simulink model "ESP_RTW"  (Simulink 8.7)
settings: Solver=ode1  SolverMode=SingleTasking  StartTime=0.0  StopTime=inf  FixedStep=0.001  RelTol=1e-3
PreLoadFcn:
  | vehicle = 'Car'; if ~length(which('cmcmd')), cmenv; end
  | ESP_RTW_bus
  | ESP_RTW_params
InitFcn:
  | vehicle = 'Car'; if ~length(which('cmcmd')), cmenv; end
  | ESP_RTW_bus
  | ESP_RTW_params
undefined symbols (not defined in the file or in its folder): Area_Front, Area_Rear, ay_max_off, ay_max_on, ay_per_mu_max_off, ay_per_mu_max_on, Brake_ratio, brake_valve_ctrl_kP, cat1mode1_higher, cat1mode1_lower, cat1mode2_higher, cat1mode2_lower, cat1mode3_higher, cat1mode3_lower, cat2mode1_higher, cat2mode1_lower, cat2mode2_higher, cat2mode2_lower, cat2mode3_higher, cat2mode3_lower, delta_vel, diff_lock_fac, diff_lock_off, diff_lock_on, ESP_ctrl_kD, ESP_ctrl_kI, ESP_ctrl_kP, ESP_ctrl_restore_kI, ESP_min_throttle_fac, f_ax, f_slip, g, higherlimit_highvel, higherlimit_lowvel, highervel_fac, highervelocity_fac, InitialConditionForIntegrator, limit_acc, limit_selectlow, limit_starting, limit_vdiff, locktime_throttle, lowerlimit_highvel, lowerlimit_lowvel, lowervel_fac, lowervelocity_fac, min_throttle, MPS2KMPH, MSR_ctrl_kD, MSR_ctrl_kI, MSR_ctrl_kP, MSR_min_throttle_fac, PID_kD_sideslip, PID_kD_yawrate, PID_kI_sideslip, PID_kI_yawrate, PID_kP_sideslip, PID_kP_yawrate, RADpS2RpM, rBrake ... (+37)
libraries: CarMaker4SL x133, simulink x47, simulink_extras x6
(part 1 of 4)
Description:
  | CarMaker Plug-in Model Target
settings Model: Creator=IPG  LastModifiedBy=IPG
settings DataIOCC: SignalLoggingSaveFormat=ModelDataLogs
settings OptimizationCC: ExpressionDepthLimit=2147483647
settings DebuggingCC: FcnCallInpInsideContextMsg=UseLocalSettings  StateNameClashWarn=warning
settings HardwareCC: TargetHWDeviceType=32-bit Generic  ProdEqTarget=off
settings RTWCC: SystemTargetFile=CarMaker.tlc  TemplateMakefile=CarMaker_unix-win64.tmf  Description=CarMaker Plug-in Model Target
settings CodeAppCC: MaxIdLength=63
settings STFCustomTargetCC: ModelReferenceCompliant=off  GeneratePreprocessorConditionals=Disable all  MultiInstanceERTCode=on  CodeInterfacePackaging=Reusable function  CPPClassGenCompliant=on  GRTInterface=off  GenerateAllocFcn=on  SystemTargetFile=CarMaker.tlc
settings GRTTargetCC: ModelReferenceCompliant=off  ParMdlRefBuildCompliant=off  CompOptLevelCompliant=off  ConcurrentExecutionCompliant=off  CombineOutputUpdateFcns=off  MatFileLogging=off  MultiInstanceERTCode=on  CodeInterfacePackaging=Reusable function  GenerateAllocFcn=on  UseToolchainInfoCompliant=off  ExtModeMexFile=noextcomm  RTWCAPISignals=on  RTWCAPIParams=on
settings CustomProperty: DataType=string  Value=..
settings EnumStrPairs: String=Car

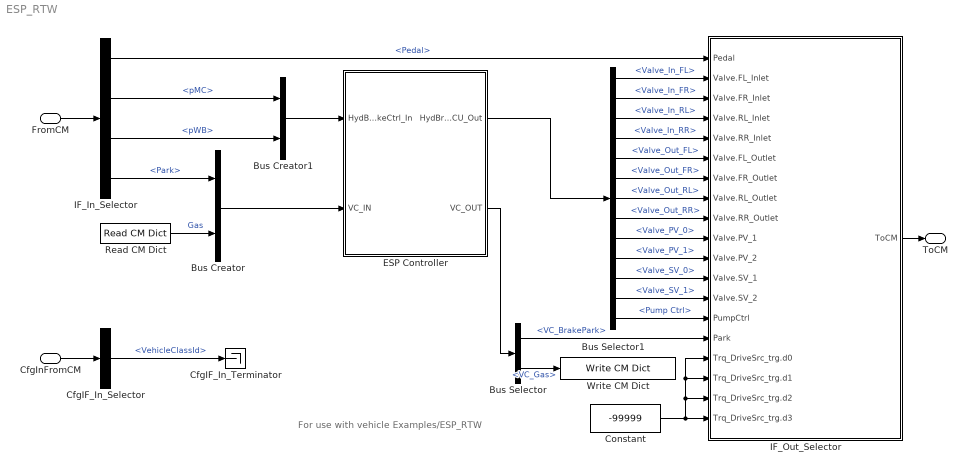
== system ESP_RTW ==
  note: For use with vehicle Examples/ESP_RTW
  FromCM : Inport  OutDataTypeStr=Bus: cmHydBrakeControlIn
  CfgInFromCM : Inport  Port=2  OutDataTypeStr=Bus: cmHydBrakeControlCfgIn
  Bus Creator : BusCreator  Inputs=2
  Bus Creator1 : BusCreator  Inputs=2
  Bus Selector : BusSelector  OutputSignals=VC_BrakePark,VC_Gas
  Bus Selector1 : BusSelector  OutputSignals=Brake Valves.Valve_In_FL,Brake Valves.Valve_In_FR,Brake Valves.Valve_In_RL,Brake Valves.Valve_In_RR,Brake Valves.Valve_Out_FL,Brake Valves.Valve_Out_FR,Brake Valves.Valve_Out_RL,Brake Valves.Valve_Out_RR,Pilot Valves.Valve_PV_0,Pilot Valves.Valve_PV_1,Suction Valves.Valve_SV_0,Suction Valves.Valve_SV_1,Pump Ctrl
  CfgIF_In_Selector : BusSelector  OutputSignals=VehicleClassId
  CfgIF_In_Terminator : Terminator
  Constant : Constant  Value=-99999
  ESP Controller : Subsystem  TreatAsAtomicUnit=on
  IF_In_Selector : BusSelector  OutputSignals=Pedal,pMC,pWB,Park
  IF_Out_Selector : Subsystem  mask(Signal Selection){}
      mask help: Signal Selection Block
      settings: OpenFcn=cmSignalSelect('SignalSelection_CB',gcb)
  Read CM Dict : CarMaker4SL/Read CM Dict  xname=VC.Gas  xsync=off
  Write CM Dict : CarMaker4SL/Write CM Dict  xname=PT.ECU.Load_lim_max  xsync=off
  ToCM : Outport  OutDataTypeStr=Bus: cmHydBrakeControlOut
  wires:
  FromCM/1 -> IF_In_Selector/1
  IF_Out_Selector/1(ToCM) -> ToCM/1
  CfgInFromCM/1 -> CfgIF_In_Selector/1
  CfgIF_In_Selector/1 -> CfgIF_In_Terminator/1  "<VehicleClassId>"
  IF_In_Selector/1 -> IF_Out_Selector/1(Pedal)  "<Pedal>"
  Bus Creator/1 -> ESP Controller/2(VC_IN)
  Bus Selector/2 -> Write CM Dict/1  "<VC_Gas>"
  Bus Selector/1 -> IF_Out_Selector/15(Park)  "<VC_BrakePark>"
  Read CM Dict/1 -> Bus Creator/2  "Gas"
  IF_In_Selector/4 -> Bus Creator/1  "<Park>"
  Bus Selector1/1 -> IF_Out_Selector/2(Valve.FL_Inlet)  "<Valve_In_FL>"
  Bus Selector1/2 -> IF_Out_Selector/3(Valve.FR_Inlet)  "<Valve_In_FR>"
  Bus Selector1/3 -> IF_Out_Selector/4(Valve.RL_Inlet)  "<Valve_In_RL>"
  Bus Selector1/4 -> IF_Out_Selector/5(Valve.RR_Inlet)  "<Valve_In_RR>"
  Bus Selector1/5 -> IF_Out_Selector/6(Valve.FL_Outlet)  "<Valve_Out_FL>"
  Bus Selector1/6 -> IF_Out_Selector/7(Valve.FR_Outlet)  "<Valve_Out_FR>"
  Bus Selector1/7 -> IF_Out_Selector/8(Valve.RL_Outlet)  "<Valve_Out_RL>"
  Bus Selector1/8 -> IF_Out_Selector/9(Valve.RR_Outlet)  "<Valve_Out_RR>"
  Bus Selector1/9 -> IF_Out_Selector/10(Valve.PV_1)  "<Valve_PV_0>"
  Bus Selector1/10 -> IF_Out_Selector/11(Valve.PV_2)  "<Valve_PV_1>"
  Bus Selector1/11 -> IF_Out_Selector/12(Valve.SV_1)  "<Valve_SV_0>"
  Bus Selector1/12 -> IF_Out_Selector/13(Valve.SV_2)  "<Valve_SV_1>"
  Bus Selector1/13 -> IF_Out_Selector/14(PumpCtrl)  "<Pump Ctrl>"
  ESP Controller/1(HydBrakeCU_Out) -> Bus Selector1/1
  ESP Controller/2(VC_OUT) -> Bus Selector/1
  Bus Creator1/1 -> ESP Controller/1(HydBrakeCtrl_In)
  IF_In_Selector/2 -> Bus Creator1/1  "<pMC>"
  IF_In_Selector/3 -> Bus Creator1/2  "<pWB>"
  Constant/1 -> IF_Out_Selector/19(Trq_DriveSrc_trg.d3), IF_Out_Selector/18(Trq_DriveSrc_trg.d2), IF_Out_Selector/17(Trq_DriveSrc_trg.d1), IF_Out_Selector/16(Trq_DriveSrc_trg.d0)

== system ESP_RTW/ESP Controller ==
  HydBrakeCtrl_In : Inport
  VC_IN : Inport  Port=2
  ESP General System : Subsystem
  ESP Input Signals : Subsystem
  Ideal Input Signals : Subsystem
  Output Signals ESP : Subsystem
  User Input Signals : Subsystem
  Vehicle Input Parameter : Subsystem
  HydBrakeCU_Out : Outport
  VC_OUT : Outport  Port=2
  wires:
  Ideal Input Signals/1(Ideal_In) -> ESP General System/4(Ideal_In)
  Vehicle Input Parameter/1(Vehicle Param) -> ESP General System/3(Vehicle Input Params)
  User Input Signals/1(User_In) -> ESP General System/2(User Input Signals)
  ESP General System/2(VC_OUT) -> VC_OUT/1
  VC_IN/1 -> ESP General System/5(VC_IN)
  ESP Input Signals/1(ESP Signals) -> ESP General System/1(ESP Input Signals)
  HydBrakeCtrl_In/1 -> ESP Input Signals/1(HydBrakeCtrl_In)
  Output Signals ESP/1(HydBrakeCU_Out) -> HydBrakeCU_Out/1
  ESP General System/1(ESP Out) -> Output Signals ESP/1(ESP Out)

== system ESP_RTW/IF_Out_Selector ==
  Pedal : Inport
  Valve.FL_Inlet : Inport  Port=2
  Valve.FR_Inlet : Inport  Port=3
  Valve.RL_Inlet : Inport  Port=4
  Valve.RR_Inlet : Inport  Port=5
  Valve.FL_Outlet : Inport  Port=6
  Valve.FR_Outlet : Inport  Port=7
  Valve.RL_Outlet : Inport  Port=8
  Valve.RR_Outlet : Inport  Port=9
  Valve.PV_1 : Inport  Port=10
  Valve.PV_2 : Inport  Port=11
  Valve.SV_1 : Inport  Port=12
  Valve.SV_2 : Inport  Port=13
  PumpCtrl : Inport  Port=14
  Park : Inport  Port=15
  Trq_DriveSrc_trg.d0 : Inport  Port=16
  Trq_DriveSrc_trg.d1 : Inport  Port=17
  Trq_DriveSrc_trg.d2 : Inport  Port=18
  Trq_DriveSrc_trg.d3 : Inport  Port=19
  BooSignal : Constant  Value=0
  RateTransition : RateTransition  OutPortSampleTime=str2num(get_param(bdroot,'FixedStep'))
  Trq_BrakeReg_trg : BusCreator  Inputs=4
  Trq_BrakeReg_trg.FL : Constant  Value=0
  Trq_BrakeReg_trg.FR : Constant  Value=0
  Trq_BrakeReg_trg.RL : Constant  Value=0
  Trq_BrakeReg_trg.RR : Constant  Value=0
  Trq_DriveSrc_trg : BusCreator  Inputs=4
  Valve : BusCreator  Inputs=16
  Valve.V_{1..4} (4 alike) : Constant  Value=0
  cmHydBrakeControlOut : BusCreator  Inputs=7
  ToCM : Outport
  wires:
  Park/1 -> cmHydBrakeControlOut/2  "Park"
  PumpCtrl/1 -> cmHydBrakeControlOut/6  "PumpCtrl"
  Valve.SV_2/1 -> Valve/12  "SV_2"
  Valve.SV_1/1 -> Valve/11  "SV_1"
  Valve.PV_2/1 -> Valve/10  "PV_2"
  Valve.PV_1/1 -> Valve/9  "PV_1"
  Valve.RR_Outlet/1 -> Valve/8  "RR_Outlet"
  Valve.RL_Outlet/1 -> Valve/7  "RL_Outlet"
  Valve.FR_Outlet/1 -> Valve/6  "FR_Outlet"
  Valve.FL_Outlet/1 -> Valve/5  "FL_Outlet"
  Valve.RR_Inlet/1 -> Valve/4  "RR_Inlet"
  Valve.RL_Inlet/1 -> Valve/3  "RL_Inlet"
  Valve.FR_Inlet/1 -> Valve/2  "FR_Inlet"
  Valve.FL_Inlet/1 -> Valve/1  "FL_Inlet"
  Pedal/1 -> cmHydBrakeControlOut/1  "Pedal"
  BooSignal/1 -> cmHydBrakeControlOut/7  "BooSignal"
  Valve.V_4/1 -> Valve/16  "V_4"
  Valve.V_3/1 -> Valve/15  "V_3"
  Valve.V_2/1 -> Valve/14  "V_2"
  Valve.V_1/1 -> Valve/13  "V_1"
  Valve/1 -> cmHydBrakeControlOut/5  "Valve"
  Trq_DriveSrc_trg/1 -> cmHydBrakeControlOut/4  "Trq_DriveSrc_trg"
  Trq_BrakeReg_trg.RR/1 -> Trq_BrakeReg_trg/4  "RR"
  Trq_BrakeReg_trg.RL/1 -> Trq_BrakeReg_trg/3  "RL"
  Trq_BrakeReg_trg.FR/1 -> Trq_BrakeReg_trg/2  "FR"
  Trq_BrakeReg_trg.FL/1 -> Trq_BrakeReg_trg/1  "FL"
  Trq_BrakeReg_trg/1 -> cmHydBrakeControlOut/3  "Trq_BrakeReg_trg"
  cmHydBrakeControlOut/1 -> RateTransition/1
  RateTransition/1 -> ToCM/1
  Trq_DriveSrc_trg.d0/1 -> Trq_DriveSrc_trg/1  "d0"
  Trq_DriveSrc_trg.d1/1 -> Trq_DriveSrc_trg/2  "d1"
  Trq_DriveSrc_trg.d2/1 -> Trq_DriveSrc_trg/3  "d2"
  Trq_DriveSrc_trg.d3/1 -> Trq_DriveSrc_trg/4  "d3"

== system ESP_RTW/ESP Controller/ESP General System ==
  ESP Input Signals : Inport
  User Input Signals : Inport  Port=2
  Vehicle Input Params : Inport  Port=3
  Ideal_In : Inport  Port=4
  VC_IN : Inport  Port=5
  ABS : Subsystem
  ASR : Subsystem
  Bus Creator : BusCreator  Inputs=6
  Bus Creator2 : BusCreator  Inputs=5
  Bus Creator3 : BusCreator  Inputs=6
  Bus Creator4 : BusCreator  Inputs=4
  ESP : Subsystem
  HSA : Subsystem
  Master Controller : Subsystem
  Signal Handling : Subsystem
  ESP Out : Outport
  VC_OUT : Outport  Port=2
  wires:
  HSA/2(BrakePark_Out) -> Master Controller/8(HSA Bus)  "BrakePark"
  HSA/1(HSA On) -> Master Controller/7(HSA On)
  Signal Handling/4(Signal Bus HSA) -> HSA/1(HSA Signal Bus)
  Signal Handling/3(Signal Bus ABS) -> ABS/1(ABS Signal Bus)
  Signal Handling/2(Signal Bus ASR) -> ASR/1(ASR Signal Bus)
  Signal Handling/1(Signal Bus ESP) -> ESP/1(ESP Signal Bus)
  Master Controller/7(VC_Out) -> VC_OUT/1  "VC_Out"
  Ideal_In/1 -> ASR/2(Ideal_In), ESP/2(Ideal_In), ABS/2(Ideal_In), HSA/2(Ideal_In)
  Master Controller/6(Diff_Torque) -> Bus Creator/6  "Diff_Torque"
  ASR/7(Diff_Torque) -> Bus Creator3/6  "Diff_Torque"
  Vehicle Input Params/1 -> ABS/3(Vehicle Params), ASR/3(Vehicle Params), ESP/3(Vehicle Params), Signal Handling/2(Vehicle Params)
  VC_IN/1 -> Master Controller/10(VC In)
  User Input Signals/1 -> ABS/4(User_In), ASR/4(User_In), ESP/4(User_In), Master Controller/9(User In)
  Bus Creator4/1 -> Master Controller/6(ABS Bus)  "ABS Bus"
  ABS/5(Pump Ctrl) -> Bus Creator4/4  "Pump Ctrl"
  ABS/4(Brake Valves) -> Bus Creator4/3  "Brake Valves"
  ABS/3(Suction Valves) -> Bus Creator4/2  "Suction Valves"
  ABS/2(Pilot Valves) -> Bus Creator4/1  "Pilot Valves"
  ASR/6(Gas_out) -> Bus Creator3/5  "Gas_Out"
  ASR/5(Pump Ctrl) -> Bus Creator3/4  "Pump Ctrl"
  ASR/4(Brake Valves) -> Bus Creator3/3  "Brake Valves"
  ASR/3(Suction Valves) -> Bus Creator3/2  "Suction Valves"
  ASR/2(Pilot Valves) -> Bus Creator3/1  "Pilot Valves"
  Master Controller/5(Pump Ctrl) -> Bus Creator/5  "Pump Ctrl"
  Master Controller/4(Suction Valves) -> Bus Creator/4  "Suction Valves"
  Master Controller/3(Pilot Valves) -> Bus Creator/3  "Pilot Valves"
  Master Controller/2(Brake Valves) -> Bus Creator/2  "Brake Valves"
  Master Controller/1(ECU Flags) -> Bus Creator/1  "ECU Flags"
  Bus Creator3/1 -> Master Controller/4(ASR Bus)  "ASR Bus"
  ABS/1(ABS On) -> Master Controller/5(ABS On)  "ABS On"
  ASR/1(ASR On) -> Master Controller/3(ASR On)  "ASR On"
  Bus Creator2/1 -> Master Controller/2(ESP Bus)  "ESP Bus"
  ESP/6(Gas_Out) -> Bus Creator2/5  "Gas_Out"
  ESP/5(Pump Ctrl) -> Bus Creator2/4  "Pump Ctrl"
  ESP/4(Brake Valves) -> Bus Creator2/3  "Brake Valves"
  ESP/3(Suction Valves) -> Bus Creator2/2  "Suction Valves"
  ESP/2(Pilot Valves) -> Bus Creator2/1  "Pilot Valves"
  ESP/1(ESP On) -> Master Controller/1(ESP On)  "ESP On"
  ESP Input Signals/1 -> Signal Handling/1(ESP In)
  Bus Creator/1 -> ESP Out/1

== system ESP_RTW/ESP Controller/ESP Input Signals ==
  HydBrakeCtrl_In : Inport
  " " : simulink_extras/Transformations/Radians to Degrees
  "   " : simulink_extras/Transformations/Radians to Degrees
  Bus Creator1 : BusCreator  Inputs=18
  Bus Selector : BusSelector  OutputSignals=Omega_B z,Acc_B y,Acc_B x
  Bus Selector1 : BusSelector  OutputSignals=pMC,pWB.FL,pWB.FR,pWB.RL,pWB.RR
  Car InertialSensor : CarMaker4SL/Car InertialSensor  xname=YRS
  Constant : Constant  Value=0
  Gain : Gain  Gain=100  SaturateOnIntegerOverflow=on  OutDataTypeStr=Inherit: Same as input  ParamDataTypeStr=Inherit: Same as input
  Gain{1..5,11} (6 alike) : Gain  Gain=RADpS2RpM  SaturateOnIntegerOverflow=on  OutDataTypeStr=Inherit: Same as input  ParamDataTypeStr=Inherit: Same as input
  Gain{6,9..10,12..15} (7 alike) : Gain  SaturateOnIntegerOverflow=on  OutDataTypeStr=Inherit: Same as input  ParamDataTypeStr=Inherit: Same as input
  Gain7 : Gain  Gain=1/g  SaturateOnIntegerOverflow=on  OutDataTypeStr=Inherit: Same as input  ParamDataTypeStr=Inherit: Same as input
  Gain8 : Gain  Gain=1/g  SaturateOnIntegerOverflow=on  OutDataTypeStr=Inherit: Same as input  ParamDataTypeStr=Inherit: Same as input
  Read CM Dict1 : CarMaker4SL/Read CM Dict  xname=Car.WheelSpd_FL  xsync=off
  Read CM Dict10 : CarMaker4SL/Read CM Dict  xname=PT.Clutch.rotv_out  xsync=off
  Read CM Dict11 : CarMaker4SL/Read CM Dict  xname=Steer.WhlAng  xsync=off
  Read CM Dict12 : CarMaker4SL/Read CM Dict  xname=PT.Engine.Trq  xsync=off
  Read CM Dict15 : CarMaker4SL/Read CM Dict  xname=PT.GearBox.GearNo  xsync=off
  Read CM Dict2 : CarMaker4SL/Read CM Dict  xname=Car.WheelSpd_FR  xsync=off
  Read CM Dict3 : CarMaker4SL/Read CM Dict  xname=Car.WheelSpd_RL  xsync=off
  Read CM Dict4 : CarMaker4SL/Read CM Dict  xname=Car.WheelSpd_RR  xsync=off
  Read CM Dict7 : CarMaker4SL/Read CM Dict  xname=PT.Engine.rotv  xsync=off
  Read CM Dict9 : CarMaker4SL/Read CM Dict  xname=VC.Gas  xsync=off
  Relational Operator : RelationalOperator  Operator=<  OutDataTypeStr=boolean
  Stop Simulation : Stop
  ESP Signals : Outport
  wires:
  Gain9/1 -> Bus Creator1/9  "Engine crankshaft output torque [Nm]"
  Gain13/1 -> Bus Creator1/14  "GearState [-]"
  " "/1 -> Bus Creator1/13  "Steering Wheel Angle [deg]"
  Gain11/1 -> Bus Creator1/12  "Torque Converter Speed [rpm]"
  Gain10/1 -> Bus Creator1/10  "Master Cylinder Pressure [bar]"
  Gain8/1 -> Bus Creator1/7  "Sensor Longitudinal acceleration [g]"
  Gain7/1 -> Bus Creator1/6  "Sensor Lateral acceleration [g]"
  "   "/1 -> Bus Creator1/5  "Sensor YawRate [degs]"
  Gain4/1 -> Bus Creator1/4  "WheelSpd RR [rpm]"
  Gain5/1 -> Bus Creator1/3  "WheelSpd RL [rpm]"
  Gain3/1 -> Bus Creator1/2  "WheelSpd FR [rpm]"
  Gain2/1 -> Bus Creator1/1  "WheelSpd FL [rpm]"
  Read CM Dict15/1 -> Gain13/1  "GearNumber [-]"
  Gain1/1 -> Bus Creator1/8  "Engine Speed [rpm]"
  Bus Selector/1 -> "   "/1  "<Omega_B z>"
  Bus Selector/3 -> Gain8/1  "<Acc_B x>"
  Car InertialSensor/2 -> Bus Selector/1
  Read CM Dict11/1 -> " "/1  "Steering Angle [rad]"
  Read CM Dict10/1 -> Gain11/1  "Clucth OutShaft [rad/s]"
  Read CM Dict9/1 -> Gain/1  "Accelerator pedal [-]"
  Bus Selector1/1 -> Gain10/1  "<pMC>"
  Read CM Dict1/1 -> Gain2/1  "WheelSpd FL [rad]/s]"
  Read CM Dict2/1 -> Gain3/1  "WheelSpd FR [rad/s]"
  Read CM Dict3/1 -> Gain5/1  "WheelSpd RL [rad/s]"
  Bus Selector/2 -> Gain7/1  "<Acc_B y>"
  Read CM Dict4/1 -> Gain4/1  "WheelSpd RR [rad/s]"
  Gain/1 -> Bus Creator1/11  "Throttle Valve Position [%]"
  Read CM Dict12/1 -> Gain9/1  "Engine Torque [Nm]"
  Read CM Dict7/1 -> Gain1/1  "Engine RotVel [rad/s]"
  Bus Creator1/1 -> ESP Signals/1
  Bus Selector1/5 -> Gain15/1  "<RR>"
  Bus Selector1/4 -> Gain14/1  "<RL>"
  Bus Selector1/3 -> Gain12/1  "<FR>"
  Bus Selector1/2 -> Gain6/1  "<FL>"
  Gain6/1 -> Bus Creator1/15  "Cylinder Pressure FL [bar]"
  Gain12/1 -> Bus Creator1/16  "Cylinder Pressure FR [bar]"
  Gain14/1 -> Bus Creator1/17  "Cylinder Pressure RL [bar]"
  Gain15/1 -> Bus Creator1/18  "Cylinder Pressure RR [bar]"
  Relational Operator/1 -> Stop Simulation/1
  Car InertialSensor/1 -> Relational Operator/1
  Constant/1 -> Relational Operator/2
  HydBrakeCtrl_In/1 -> Bus Selector1/1

== system ESP_RTW/ESP Controller/Ideal Input Signals ==
  Bus Creator1 : BusCreator  Inputs=8
  Bus Creator2 : BusCreator  Inputs=4
  Bus Creator3 : BusCreator  Inputs=2
  Bus Creator4 : BusCreator  Inputs=2
  Bus Creator5 : BusCreator  Inputs=3
  Bus Creator6 : BusCreator  Inputs=2
  Read CM Dict1 : CarMaker4SL/Read CM Dict  xname=Car.Pitch  xsync=off
  Read CM Dict10 : CarMaker4SL/Read CM Dict  xname=Car.FzRL  xsync=off
  Read CM Dict11 : CarMaker4SL/Read CM Dict  xname=Car.YawRate  xsync=off
  Read CM Dict13 : CarMaker4SL/Read CM Dict  xname=Car.CRL.Trq_T2W  xsync=off
  Read CM Dict14 : CarMaker4SL/Read CM Dict  xname=Car.LongSlipRL  xsync=off
  Read CM Dict16 : CarMaker4SL/Read CM Dict  xname=Car.CRR.Trq_T2W  xsync=off
  Read CM Dict17 : CarMaker4SL/Read CM Dict  xname=Car.FzRR  xsync=off
  Read CM Dict19 : CarMaker4SL/Read CM Dict  xname=Car.LongSlipRR  xsync=off
  Read CM Dict2 : CarMaker4SL/Read CM Dict  xname=Car.v  xsync=off
  Read CM Dict3 : CarMaker4SL/Read CM Dict  xname=Car.muRoadFR  xsync=off
  Read CM Dict4 : CarMaker4SL/Read CM Dict  xname=Car.muRoadRL  xsync=off
  Read CM Dict5 : CarMaker4SL/Read CM Dict  xname=Car.SideSlipAngle  xsync=off
  Read CM Dict6 : CarMaker4SL/Read CM Dict  xname=Car.muRoadFL  xsync=off
  Read CM Dict7 : CarMaker4SL/Read CM Dict  xname=Car.muRoadRR  xsync=off
  Read CM Dict8 : CarMaker4SL/Read CM Dict  xname=Car.vx  xsync=off
  Read CM Dict9 : CarMaker4SL/Read CM Dict  xname=Car.vy  xsync=off
  Ideal_In : Outport
  wires:
  Bus Creator6/1 -> Bus Creator1/8  "Ideal_Slip"
  Bus Creator4/1 -> Bus Creator1/7  "Ideal_Fz"
  Bus Creator3/1 -> Bus Creator1/6  "Idea_Trq2W"
  Bus Creator2/1 -> Bus Creator1/5  "Ideal_mu"
  Read CM Dict11/1 -> Bus Creator1/4  "Ideal_YawRate"
  Read CM Dict19/1 -> Bus Creator6/2  "Ideal_SlipRR"
  Read CM Dict14/1 -> Bus Creator6/1  "Ideal_SlipRL"
  Read CM Dict9/1 -> Bus Creator5/3  "Ideal_Velocity_y"
  Bus Creator5/1 -> Bus Creator1/2  "Ideal_Velocity"
  Read CM Dict8/1 -> Bus Creator5/2  "Ideal_Velocity_x"
  Read CM Dict2/1 -> Bus Creator5/1  "Ideal_Velocity"
  Read CM Dict5/1 -> Bus Creator1/3  "Ideal_SideSlipAngle"
  Read CM Dict1/1 -> Bus Creator1/1  "Ideal_Pitch"
  Bus Creator1/1 -> Ideal_In/1
  Read CM Dict7/1 -> Bus Creator2/4  "Ideal_muRR"
  Read CM Dict4/1 -> Bus Creator2/3  "Ideal_muRL"
  Read CM Dict3/1 -> Bus Creator2/2  "Ideal_muFR"
  Read CM Dict6/1 -> Bus Creator2/1  "Ideal_muFL"
  Read CM Dict13/1 -> Bus Creator3/1  "Ideal_Trq2WRL"
  Read CM Dict16/1 -> Bus Creator3/2  "Ideal_Trq2WRR"
  Read CM Dict10/1 -> Bus Creator4/1  "Ideal_FzRL"
  Read CM Dict17/1 -> Bus Creator4/2  "Ideal_FzRR"

== system ESP_RTW/ESP Controller/Output Signals ESP ==
  ESP Out : Inport
  Bus Creator : BusCreator  Inputs=4
  Bus Selector : BusSelector  OutputSignals=ECU Flags,Brake Valves,Pilot Valves,Suction Valves,Pump Ctrl,Diff_Torque
  Bus Selector1 : BusSelector  OutputSignals=ESP On,ASR On,ABS On,HSA On
  Bus Selector2 : BusSelector  OutputSignals=ASR On,MSR On,BMR On
  Bus Selector4 : BusSelector  OutputSignals=FrontDiff_Torque
  Data Type Conversion : DataTypeConversion
  Define CM Dict1 : CarMaker4SL/Define CM Dict  xname=ESP.ASR.MSR.active  xmono=off  xtype=Char  xdvaplace=VC  xnstates=2  xfirststate=0  xinitial=0
  Define CM Dict10 : CarMaker4SL/Define CM Dict  xname=ESP.ESP.active  xmono=off  xtype=Char  xdvaplace=VC  xnstates=2  xfirststate=0  xinitial=0
  Define CM Dict2 : CarMaker4SL/Define CM Dict  xname=ESP.ASR.BMR.active  xmono=off  xtype=Char  xdvaplace=VC  xnstates=2  xfirststate=0  xinitial=0
  Define CM Dict3 : CarMaker4SL/Define CM Dict  xname=ESP.ASR.active  xmono=off  xtype=Char  xdvaplace=VC  xnstates=2  xfirststate=0  xinitial=0
  Define CM Dict4 : CarMaker4SL/Define CM Dict  xname=ESP.HSA.active  xmono=off  xtype=Char  xdvaplace=VC  xnstates=2  xfirststate=0  xinitial=0
  Define CM Dict6 : CarMaker4SL/Define CM Dict  xname=ESP.ESP.lamp  xmono=off  xtype=Char  xdvaplace=VC  xnstates=2  xfirststate=0  xinitial=0
  Define CM Dict9 : CarMaker4SL/Define CM Dict  xname=ESP.ABS.active  xmono=off  xtype=Char  xdvaplace=VC  xnstates=2  xfirststate=0  xinitial=0
  Logical Operator : Logic  Operator=OR  AllPortsSameDT=off  OutDataTypeStr=boolean
  Read CM Dict3 : CarMaker4SL/Read CM Dict  xname=ESP.User.ESP_off  xsync=off
  Write CM Dict12 : CarMaker4SL/Write CM Dict  xname=ESP.ASR.MSR.active  xsync=off
  Write CM Dict13 : CarMaker4SL/Write CM Dict  xname=ESP.ASR.BMR.active  xsync=off
  Write CM Dict15 : CarMaker4SL/Write CM Dict  xname=ESP.ASR.active  xsync=off
  Write CM Dict17 : CarMaker4SL/Write CM Dict  xname=ESP.ABS.active  xsync=off
  Write CM Dict18 : CarMaker4SL/Write CM Dict  xname=ESP.ESP.active  xsync=off
  Write CM Dict19 : CarMaker4SL/Write CM Dict  xname=PT.Gen.DL.FDiff.DVA.Trq_A2B  xsync=off
  Write CM Dict20 : CarMaker4SL/Write CM Dict  xname=ESP.HSA.active  xsync=off
  Write CM Dict21 : CarMaker4SL/Write CM Dict  xname=ESP.ESP.lamp  xsync=off
  HydBrakeCU_Out : Outport
  wires:
  ESP Out/1 -> Bus Selector/1
  Bus Selector/1 -> Bus Selector1/1  "<ECU Flags>"
  Bus Selector1/2 -> Bus Selector2/1  "<ASR On>"
  Bus Selector1/1 -> Logical Operator/2, Write CM Dict18/1  "<ESP On>"
  Bus Selector1/3 -> Write CM Dict17/1  "<ABS On>"
  Bus Selector2/1 -> Write CM Dict15/1  "<ASR On>"
  Bus Selector2/2 -> Write CM Dict12/1  "<MSR On>"
  Bus Selector2/3 -> Write CM Dict13/1  "<BMR On>"
  Bus Selector4/1 -> Write CM Dict19/1  "<FrontDiff_Torque>"
  Bus Selector/6 -> Bus Selector4/1  "<Diff_Torque>"
  Bus Selector1/4 -> Write CM Dict20/1  "<HSA On>"
  Logical Operator/1 -> Data Type Conversion/1
  Read CM Dict3/1 -> Logical Operator/1
  Data Type Conversion/1 -> Write CM Dict21/1
  Bus Selector/2 -> Bus Creator/1  "<Brake Valves>"
  Bus Selector/3 -> Bus Creator/2  "<Pilot Valves>"
  Bus Selector/4 -> Bus Creator/3  "<Suction Valves>"
  Bus Selector/5 -> Bus Creator/4  "<Pump Ctrl>"
  Bus Creator/1 -> HydBrakeCU_Out/1

== system ESP_RTW/ESP Controller/User Input Signals ==
  note: User_Drive: 1 = Front; 2 = Rear; 3 = AllWheel
  Bus Creator1 : BusCreator  Inputs=5
  Bus Creator2 : BusCreator  Inputs=5
  Bus Creator3 : BusCreator  Inputs=2
  Bus Creator4 : BusCreator  Inputs=2
  Define CM Dict1 : CarMaker4SL/Define CM Dict  xname=ESP.User.ESP_off  xmono=off  xtype=Char  xdvaplace=IO_Out  xnstates=2  xfirststate=0  xinitial=0
  Define CM Dict10 : CarMaker4SL/Define CM Dict  xname=ESP.User.HSA_off  xmono=off  xtype=Char  xdvaplace=IO_Out  xnstates=2  xfirststate=0  xinitial=0
  Define CM Dict11 : CarMaker4SL/Define CM Dict  xname=ESP.User.oneWheel_on  xmono=off  xtype=Char  xdvaplace=IO_Out  xnstates=2  xfirststate=0  xinitial=0
  Define CM Dict2 : CarMaker4SL/Define CM Dict  xname=ESP.User.ASR_off  xmono=off  xtype=Char  xdvaplace=IO_Out  xnstates=2  xfirststate=0  xinitial=0
  Define CM Dict3 : CarMaker4SL/Define CM Dict  xname=ESP.User.ABS_off  xmono=off  xtype=Char  xdvaplace=IO_Out  xnstates=2  xfirststate=0  xinitial=0
  Define CM Dict4 : CarMaker4SL/Define CM Dict  xname=ESP.User.ESP_all_off  xmono=off  xtype=Char  xdvaplace=IO_Out  xnstates=2  xfirststate=0  xinitial=0
  Define CM Dict5 : CarMaker4SL/Define CM Dict  xname=ESP.User.Drive  xmono=off  xtype=Char  xdvaplace=IO_Out  xnstates=3  xfirststate=1  xinitial=1
  Define CM Dict6 : CarMaker4SL/Define CM Dict  xname=ESP.User.SideSlip_estimator_on  xmono=off  xtype=Char  xdvaplace=IO_Out  xnstates=2  xfirststate=0  xinitial=0
  Define CM Dict7 : CarMaker4SL/Define CM Dict  xname=ESP.User.mue_estimator_on  xmono=off  xtype=Char  xdvaplace=IO_Out  xnstates=2  xfirststate=0  xinitial=0
  Define CM Dict8 : CarMaker4SL/Define CM Dict  xname=ESP.User.DiffLockDVA_on  xmono=off  xtype=Char  xdvaplace=IO_Out  xnstates=2  xfirststate=0  xinitial=0
  Define CM Dict9 : CarMaker4SL/Define CM Dict  xname=ESP.User.DiffLockDVA_Trq  xunit=Nm  xmono=off  xtype=Double4  xdvaplace=IO_Out  xnstates=2  xfirststate=0  xinitial=0
  Read CM Dict1 : CarMaker4SL/Read CM Dict  xname=ESP.User.Drive  xsync=off
  Read CM Dict10 : CarMaker4SL/Read CM Dict  xname=ESP.User.HSA_off  xsync=off
  Read CM Dict11 : CarMaker4SL/Read CM Dict  xname=ESP.User.oneWheel_on  xsync=off
  Read CM Dict2 : CarMaker4SL/Read CM Dict  xname=ESP.User.ESP_all_off  xsync=off
  Read CM Dict3 : CarMaker4SL/Read CM Dict  xname=ESP.User.ESP_off  xsync=off
  Read CM Dict4 : CarMaker4SL/Read CM Dict  xname=ESP.User.ASR_off  xsync=off
  Read CM Dict5 : CarMaker4SL/Read CM Dict  xname=ESP.User.ABS_off  xsync=off
  Read CM Dict6 : CarMaker4SL/Read CM Dict  xname=ESP.User.SideSlip_estimator_on  xsync=off
  Read CM Dict7 : CarMaker4SL/Read CM Dict  xname=ESP.User.mue_estimator_on  xsync=off
  Read CM Dict8 : CarMaker4SL/Read CM Dict  xname=ESP.User.DiffLockDVA_on  xsync=off
  Read CM Dict9 : CarMaker4SL/Read CM Dict  xname=ESP.User.DiffLockDVA_Trq  xsync=off
  User_In : Outport
  wires:
  Read CM Dict11/1 -> Bus Creator1/5  "User_oneWheel_on"
  Read CM Dict10/1 -> Bus Creator2/5  "User_Switch_HSA_off"
  Bus Creator4/1 -> Bus Creator1/4  "User_DiffLock"
  Read CM Dict9/1 -> Bus Creator4/2  "User_DiffLock_Trq"
  Read CM Dict8/1 -> Bus Creator4/1  "User_DiffLock_on"
  Bus Creator3/1 -> Bus Creator1/3  "User_estimators_on"
  Read CM Dict7/1 -> Bus Creator3/2  "User_mue_estimator_on"
  Read CM Dict6/1 -> Bus Creator3/1  "User_SideSlip_estimator_on"
  Bus Creator2/1 -> Bus Creator1/2  "User_Switch"
  Read CM Dict2/1 -> Bus Creator2/1  "User_Switch_Main_off"
  Read CM Dict3/1 -> Bus Creator2/2  "User_Switch_ESP_off"
  Read CM Dict4/1 -> Bus Creator2/3  "User_Switch_ASR_off"
  Read CM Dict5/1 -> Bus Creator2/4  "User_Switch_ABS_off"
  Bus Creator1/1 -> User_In/1
  Read CM Dict1/1 -> Bus Creator1/1  "User_Drive"

== system ESP_RTW/ESP Controller/Vehicle Input Parameter ==
  note: Note:
      | We could also use
      | the left wheel as is has
      | the same coordinate
      | as regards x-axis
      | (which interests us here)
  note: Note:
      | We could also use
      | the left wheel as is has
      | the same coordinate
      | as regards x-axis
      | (which interests us here)
  Bus Creator{,1..3} (4 alike) : BusCreator  Inputs=4
  Bus Creator4 : BusCreator  Inputs=2
  Read CM Parameter : CarMaker4SL/Read CM Parameter  xfile=TireFL  xkey=KinRollRadius  xnout=1  xdefaults=0  xmuxed=on
  Read CM Parameter1 : CarMaker4SL/Read CM Parameter  xfile=TireFR  xkey=KinRollRadius  xnout=1  xdefaults=0  xmuxed=on
  Read CM Parameter2 : CarMaker4SL/Read CM Parameter  xfile=TireRL  xkey=KinRollRadius  xnout=1  xdefaults=0  xmuxed=on
  Read CM Parameter3 : CarMaker4SL/Read CM Parameter  xfile=TireRR  xkey=KinRollRadius  xnout=1  xdefaults=0  xmuxed=on
  Read CM Parameter4 : CarMaker4SL/Read CM Parameter  xfile=Vehicle  xkey=WheelCarrier.fr.pos  xnout=1  xdefaults=0  xmuxed=on
  Read CM Parameter5 : CarMaker4SL/Read CM Parameter  xfile=Vehicle  xkey=Body.pos  xnout=1  xdefaults=0  xmuxed=on
  Read CM Parameter6 : CarMaker4SL/Read CM Parameter  xfile=Vehicle  xkey=Body.pos  xnout=1  xdefaults=0  xmuxed=on
  Read CM Parameter7 : CarMaker4SL/Read CM Parameter  xfile=Vehicle  xkey=WheelCarrier.rr.pos  xnout=1  xdefaults=0  xmuxed=on
  Read CM Parameter8 : CarMaker4SL/Read CM Parameter  xfile=Vehicle  xkey=WheelCarrier.rl.pos  xnout=2  xdefaults=0  xmuxed=off
  Read CM Parameter9 : CarMaker4SL/Read CM Parameter  xfile=Vehicle  xkey=WheelCarrier.fl.pos  xnout=2  xdefaults=0  xmuxed=off
  Steer Angle y-Data : Constant  Value=SteerAng_Out
  Steer Wheel Angle x-Data : Constant  Value=SteerWheelAng_In
  Sum3 : Sum  Inputs=+-  SaturateOnIntegerOverflow=on  InputSameDT=on  OutDataTypeStr=Inherit: Same as first input
  Sum4 : Sum  Inputs=+-  SaturateOnIntegerOverflow=on  InputSameDT=on  OutDataTypeStr=Inherit: Same as first input
  Terminator{,1..9} (10 alike) : Terminator
  z-Position of WheelCarrier FL : CarMaker4SL/Read CM Parameter  xfile=Vehicle  xkey=WheelCarrier.fl.pos  xnout=3  xdefaults=0  xmuxed=off
  z-Position of WheelCarrier FR : CarMaker4SL/Read CM Parameter  xfile=Vehicle  xkey=WheelCarrier.fr.pos  xnout=3  xdefaults=0  xmuxed=off
  z-Position of WheelCarrier RL : CarMaker4SL/Read CM Parameter  xfile=Vehicle  xkey=WheelCarrier.rl.pos  xnout=3  xdefaults=0  xmuxed=off
  z-Position of WheelCarrier RR : CarMaker4SL/Read CM Parameter  xfile=Vehicle  xkey=WheelCarrier.rr.pos  xnout=3  xdefaults=0  xmuxed=off
  Vehicle Param : Outport
  wires:
  Bus Creator4/1 -> Bus Creator1/4  "SteeringGeometry"
  Steer Wheel Angle x-Data/1 -> Bus Creator4/1  "SteerWheelAng_In"
  Steer Angle y-Data/1 -> Bus Creator4/2  "SteerAng_Out"
  z-Position of WheelCarrier RR/2 -> Terminator9/1
  z-Position of WheelCarrier RR/1 -> Terminator8/1
  z-Position of WheelCarrier RL/2 -> Terminator7/1
  z-Position of WheelCarrier RL/1 -> Terminator6/1
  z-Position of WheelCarrier FR/2 -> Terminator5/1
  z-Position of WheelCarrier FR/1 -> Terminator4/1
  z-Position of WheelCarrier RR/3 -> Bus Creator3/4  "Param_zRR"
  z-Position of WheelCarrier RL/3 -> Bus Creator3/3  "Param_zRL"
  z-Position of WheelCarrier FR/3 -> Bus Creator3/2  "Param_zFR"
  z-Position of WheelCarrier FL/3 -> Bus Creator3/1  "Param_zFL"
  Bus Creator3/1 -> Bus Creator1/3  "CarrierGeometry"
  z-Position of WheelCarrier FL/2 -> Terminator3/1
  z-Position of WheelCarrier FL/1 -> Terminator2/1
  Read CM Parameter8/1 -> Terminator1/1
  Read CM Parameter9/1 -> Terminator/1
  Read CM Parameter9/2 -> Bus Creator2/3  "Param_bF"
  Read CM Parameter8/2 -> Bus Creator2/4  "Param_bR"
  Bus Creator2/1 -> Bus Creator1/2  "VehicleGeometry"
  Read CM Parameter6/1 -> Sum3/1
  Sum3/1 -> Bus Creator2/2  "Param_aR"
  Read CM Parameter7/1 -> Sum3/2
  Sum4/1 -> Bus Creator2/1  "Param_aF"
  Read CM Parameter4/1 -> Sum4/1
  Read CM Parameter5/1 -> Sum4/2
  Read CM Parameter2/1 -> Bus Creator/3  "Param_RadiusRL"
  Read CM Parameter/1 -> Bus Creator/1  "Param_RadiusFL"
  Bus Creator/1 -> Bus Creator1/1  "TireRadius"
  Read CM Parameter3/1 -> Bus Creator/4  "Param_RadiusRR"
  Read CM Parameter1/1 -> Bus Creator/2  "Param_RadiusFR"
  Bus Creator1/1 -> Vehicle Param/1

== system ESP_RTW/ESP Controller/ESP General System/ABS ==
  note: ABS disabled when slower than v_min
  ABS Signal Bus : Inport
  Ideal_In : Inport  Port=2
  Vehicle Params : Inport  Port=3
  User_In : Inport  Port=4
  ABS ECU : Subsystem
  Bus Creator : BusCreator  Inputs=8
  Bus Creator2 : BusCreator  Inputs=2
  Bus Creator3 : BusCreator  Inputs=2
  Bus Selector3 : BusSelector  OutputSignals=ax [m/s^2],WheelSpeeds
  Bus Selector1 : BusSelector  OutputSignals=TireRadius
  Bus Selector2 : BusSelector  OutputSignals=Param_RadiusRR,Param_RadiusRL,Param_RadiusFR,Param_RadiusFL
  Bus Selector4 : BusSelector  OutputSignals=WheelSpd_RR,WheelSpd_RL,WheelSpd_FR,WheelSpd_FL
  helpsignals estimator : Subsystem
  ABS On : Outport
  Pilot Valves : Outport  Port=2
  Suction Valves : Outport  Port=3
  Brake Valves : Outport  Port=4
  Pump Ctrl : Outport  Port=5
  wires:
  Bus Selector4/1 -> ABS ECU/9(Speed_RR)  "<WheelSpd_RR>"
  Bus Selector4/2 -> ABS ECU/8(Speed_RL)  "<WheelSpd_RL>"
  Bus Selector4/3 -> ABS ECU/7(Speed_FR)  "<WheelSpd_FR>"
  Bus Selector4/4 -> ABS ECU/6(Speed_FL)  "<WheelSpd_FL>"
  Ideal_In/1 -> helpsignals estimator/2(Ideal_In)
  Bus Selector3/1 -> helpsignals estimator/3(ax)  "<ax [m/s^2]>"
  ABS Signal Bus/1 -> Bus Selector3/1
  Bus Selector1/1 -> helpsignals estimator/5(TireRadius), Bus Selector2/1  "<TireRadius>"
  Bus Selector2/1 -> ABS ECU/13(radius_RR)  "<Param_RadiusRR>"
  Bus Selector2/2 -> ABS ECU/12(radius_RL)  "<Param_RadiusRL>"
  Bus Selector2/3 -> ABS ECU/11(radius_FR)  "<Param_RadiusFR>"
  Vehicle Params/1 -> Bus Selector1/1
  Bus Selector2/4 -> ABS ECU/10(radius_FL)  "<Param_RadiusFL>"
  User_In/1 -> helpsignals estimator/1(User_In)
  Bus Creator3/1 -> Suction Valves/1
  Bus Creator2/1 -> Pilot Valves/1
  ABS ECU/14(Valve_SV_1) -> Bus Creator3/2  "Valve_SV_1"
  ABS ECU/13(Valve_SV_0) -> Bus Creator3/1  "Valve_SV_0"
  ABS ECU/12(Valve_PV_1) -> Bus Creator2/2  "Valve_PV_1"
  ABS ECU/11(Valve_PV_0) -> Bus Creator2/1  "Valve_PV_0"
  ABS ECU/9(Brake Valve_Out_RR) -> Bus Creator/8  "Valve_Out_RR"
  ABS ECU/8(Brake Valve_Out_RL) -> Bus Creator/7  "Valve_Out_RL"
  ABS ECU/7(Brake Valve_Out_FR) -> Bus Creator/6  "Valve_Out_FR"
  ABS ECU/6(Brake Valve_Out_FL) -> Bus Creator/5  "Valve_Out_FL"
  ABS ECU/5(Brake Valve_In_RR) -> Bus Creator/4  "Valve_In_RR"
  ABS ECU/4(Brake Valve_In_RL) -> Bus Creator/3  "Valve_In_RL"
  ABS ECU/3(Brake Valve_In_FR) -> Bus Creator/2  "Valve_In_FR"
  ABS ECU/2(Brake Valve_In_FL) -> Bus Creator/1  "Valve_In_FL"
  Bus Creator/1 -> Brake Valves/1
  Bus Selector3/2 -> helpsignals estimator/4(WheelSpeeds), Bus Selector4/1  "<WheelSpeeds>"
  ABS ECU/10(ABS On) -> ABS On/1
  helpsignals estimator/5(LongSlip_RR) -> ABS ECU/5(LongSlip_RR)
  ABS ECU/1(Brake Pump Ctrl) -> Pump Ctrl/1
  helpsignals estimator/4(LongSlip_RL) -> ABS ECU/4(LongSlip_RL)
  helpsignals estimator/3(LongSlip_FR) -> ABS ECU/3(LongSlip_FR)
  helpsignals estimator/2(LongSlip_FL) -> ABS ECU/2(LongSlip_FL)
  helpsignals estimator/1(vref) -> ABS ECU/1(vref)

== system ESP_RTW/ESP Controller/ESP General System/ASR ==
  ASR Signal Bus : Inport
  Ideal_In : Inport  Port=2
  Vehicle Params : Inport  Port=3
  User_In : Inport  Port=4
  BMR ECU : Subsystem
  Bus Creator : BusCreator  Inputs=4
  Bus Creator3 : BusCreator  Inputs=3
  Bus Selector3 : BusSelector  OutputSignals=Throttle Position,WheelSpeeds
  Bus Selector : BusSelector  OutputSignals=WheelSpd_FL,WheelSpd_FR,WheelSpd_RL,WheelSpd_RR
  Bus Selector1 : BusSelector  OutputSignals=TireRadius
  Bus Selector2 : BusSelector  OutputSignals=Param_RadiusFL,Param_RadiusFR,Param_RadiusRL,Param_RadiusRR
  Constant4 : Constant  Value=MPS2KMPH
  Logical Operator2 : Logic  Operator=OR  AllPortsSameDT=off
  MSR ECU : Subsystem
  Mux1 : Mux
  Product : Product  RndMeth=Zero
  Product1 : Product  RndMeth=Zero
  ASR On : Outport
  Pilot Valves : Outport  Port=2
  Suction Valves : Outport  Port=3
  Brake Valves : Outport  Port=4
  Pump Ctrl : Outport  Port=5
  Gas_out : Outport  Port=6
  Diff_Torque : Outport  Port=7
  wires:
  Constant4/1 -> Product1/2
  Ideal_In/1 -> BMR ECU/4(Ideal_In), MSR ECU/4(Ideal_In)
  Bus Selector3/1 -> MSR ECU/1(Throttle Position), BMR ECU/1(Throttle)  "<Throttle Position>"
  ASR Signal Bus/1 -> Bus Selector3/1
  Bus Selector1/1 -> Bus Selector2/1  "<TireRadius>"
  Bus Selector2/4 -> Mux1/4  "<Param_RadiusRR>"
  Bus Selector2/3 -> Mux1/3  "<Param_RadiusRL>"
  Bus Selector2/2 -> Mux1/2  "<Param_RadiusFR>"
  Vehicle Params/1 -> Bus Selector1/1
  BMR ECU/6(Diff_Torque) -> Diff_Torque/1  "Diff_Torque"
  User_In/1 -> BMR ECU/3(User_In), MSR ECU/3(User_In)
  BMR ECU/5(Pump Ctrl) -> Pump Ctrl/1
  BMR ECU/4(Suctions Valves) -> Suction Valves/1
  BMR ECU/3(Pilot Valves) -> Pilot Valves/1
  Logical Operator2/1 -> Bus Creator3/2  "ASR On"
  Bus Creator3/1 -> ASR On/1
  MSR ECU/1(Gas_out) -> Gas_out/1
  Mux1/1 -> Product/2
  Bus Creator/1 -> Product/1
  Product1/1 -> MSR ECU/2(WheelVelocity [kmph]), BMR ECU/2(WheelVelocity [kmph])
  BMR ECU/2(Brake Valves) -> Brake Valves/1
  BMR ECU/1(BMR On) -> Bus Creator3/3, Logical Operator2/2  "BMR On"
  MSR ECU/2(MSR On) -> Logical Operator2/1, Bus Creator3/1  "MSR On"
  Bus Selector3/2 -> Bus Selector/1  "<WheelSpeeds>"
  Bus Selector2/1 -> Mux1/1  "<Param_RadiusFL>"
  Bus Selector/4 -> Bus Creator/4  "<WheelSpd_RR>"
  Bus Selector/3 -> Bus Creator/3  "<WheelSpd_RL>"
  Bus Selector/2 -> Bus Creator/2  "<WheelSpd_FR>"
  Bus Selector/1 -> Bus Creator/1  "<WheelSpd_FL>"
  Product/1 -> Product1/1

== system ESP_RTW/ESP Controller/ESP General System/ESP ==
  ESP Signal Bus : Inport
  Ideal_In : Inport  Port=2
  Vehicle Params : Inport  Port=3
  User_In : Inport  Port=4
  Actuator Brake : Subsystem
  Bus Creator : BusCreator  Inputs=8
  Bus Creator1 : BusCreator  Inputs=2
  Bus Creator2 : BusCreator  Inputs=2
  Bus Selector1 : BusSelector  OutputSignals=ax [m/s^2],Throttle Position,Yaw Rate,Steer Angle,ay [m/s^2],Wheel Cylinder Pressure
  Define CM Dict : CarMaker4SL/Define CM Dict  xname=ESP.ESP.Gas_out  xmono=off  xtype=Double4  xdvaplace=None  xnstates=0  xfirststate=0  xinitial=0
  ECU : Subsystem
  Write CM Dict : CarMaker4SL/Write CM Dict  xname=ESP.ESP.Gas_out  xsync=off
  helpsignals estimator : Subsystem
  ESP On : Outport
  Pilot Valves : Outport  Port=2
  Suction Valves : Outport  Port=3
  Brake Valves : Outport  Port=4
  Pump Ctrl : Outport  Port=5
  Gas_Out : Outport  Port=6
  wires:
  Bus Selector1/5 -> ECU/7(ay)  "<ay [m/s^2]>"
  ESP Signal Bus/1 -> Bus Selector1/1
  Vehicle Params/1 -> helpsignals estimator/3(Vehicle Params), ECU/9(Vehicle Params)
  Bus Selector1/6 -> Actuator Brake/9(Wheel Cylinder Pressure)  "<Wheel Cylinder Pressure>"
  Ideal_In/1 -> helpsignals estimator/2(Ideal_In), ECU/8(Ideal_In)
  User_In/1 -> helpsignals estimator/4(User_In), ECU/10(User_In)
  Bus Creator1/1 -> Suction Valves/1
  Bus Creator2/1 -> Pilot Valves/1
  Bus Creator/1 -> Brake Valves/1
  ECU/1(Gas_out) -> Gas_Out/1, Write CM Dict/1
  Actuator Brake/14(ESP_On) -> ESP On/1  "ESP_On"
  Actuator Brake/13(PumpCtrl) -> Pump Ctrl/1  "PumpCtrl"
  Actuator Brake/12(Valve_SV_1) -> Bus Creator1/2  "Valve_SV_1"
  Actuator Brake/11(Valve_SV_0) -> Bus Creator1/1  "Valve_SV_0"
  Actuator Brake/10(Valve_PV_1) -> Bus Creator2/2  "Valve_PV_1"
  Actuator Brake/9(Valve_PV_0) -> Bus Creator2/1  "Valve_PV_0"
  Actuator Brake/8(Valve_Out_RR) -> Bus Creator/8  "Valve_Out_RR"
  Actuator Brake/7(Valve_Out_RL) -> Bus Creator/7  "Valve_Out_RL"
  Bus Selector1/3 -> ECU/3(Yaw Rate)  "<Yaw Rate>"
  Actuator Brake/6(Valve_Out_FR) -> Bus Creator/6  "Valve_Out_FR"
  Actuator Brake/5(Valve_Out_FL) -> Bus Creator/5  "Valve_Out_FL"
  Bus Selector1/2 -> ECU/2(Throttle Position)  "<Throttle Position>"
  Actuator Brake/4(Valve_In_RR) -> Bus Creator/4  "Valve_In_RR"
  Actuator Brake/3(Valve_In_RL) -> Bus Creator/3  "Valve_In_RL"
  Bus Selector1/1 -> ECU/1(ax)  "<ax [m/s^2]>"
  Actuator Brake/2(Valve_In_FR) -> Bus Creator/2  "Valve_In_FR"
  Actuator Brake/1(Valve_In_FL) -> Bus Creator/1  "Valve_In_FL"
  Bus Selector1/4 -> helpsignals estimator/1(Steer Angle), ECU/4(Steer Angle)  "<Steer Angle>"
  helpsignals estimator/2(mu) -> ECU/6(mu)
  helpsignals estimator/1(SideslipAngle) -> ECU/5(Sideslip)
  ECU/9(RR_Trq_target) -> Actuator Brake/8(RR_Trq_target)
  ECU/8(RR_active) -> Actuator Brake/7(RR_active)
  ECU/7(RL_Trq_target) -> Actuator Brake/6(RL_Trq_target)
  ECU/6(RL_active) -> Actuator Brake/5(RL_active)
  ECU/5(FR_Trq_target) -> Actuator Brake/4(FR_Trq_target)
  ECU/4(FR_active) -> Actuator Brake/3(FR_active)
  ECU/3(FL_Trq_target) -> Actuator Brake/2(FL_Trq_target)
  ECU/2(FL_active) -> Actuator Brake/1(FL_active)

== system ESP_RTW/ESP Controller/ESP General System/HSA ==
  HSA Signal Bus : Inport
  Ideal_In : Inport  Port=2
  Bus Selector2 : BusSelector  OutputSignals=Engine crankshaft output torque [Nm]
  Bus Selector1 : BusSelector  OutputSignals=Ideal_Pitch,Ideal_Velocity.Ideal_Velocity_x
  Data Type Conversion : DataTypeConversion
  Gain : Gain  Gain=-1
  Logical Operator : Logic  Inputs=3  AllPortsSameDT=off  OutDataTypeStr=boolean
  Relay : Relay  OnSwitchValue=threshold_carpitch_on  OffSwitchValue=threshold_carpitch_off
  Relay1 : Relay  OnSwitchValue=threshold_velocity_on  OffSwitchValue=threshold_velocity_off  OnOutputValue=0  OffOutputValue=1
  Relay2 : Relay  OnSwitchValue=threshold_eng_trq_on  OffSwitchValue=threshold_eng_trq_off  OnOutputValue=0  OffOutputValue=1
  HSA On : Outport
  BrakePark_Out : Outport  Port=2
  wires:
  Bus Selector2/1 -> Relay2/1  "<Engine crankshaft output torque [Nm]>"
  HSA Signal Bus/1 -> Bus Selector2/1
  Data Type Conversion/1 -> BrakePark_Out/1, HSA On/1
  Logical Operator/1 -> Data Type Conversion/1
  Relay/1 -> Logical Operator/2
  Relay1/1 -> Logical Operator/3
  Relay2/1 -> Logical Operator/1
  Bus Selector1/2 -> Relay1/1  "<Ideal_Velocity_x>"
  Gain/1 -> Relay/1
  Bus Selector1/1 -> Gain/1  "<Ideal_Pitch>"
  Ideal_In/1 -> Bus Selector1/1

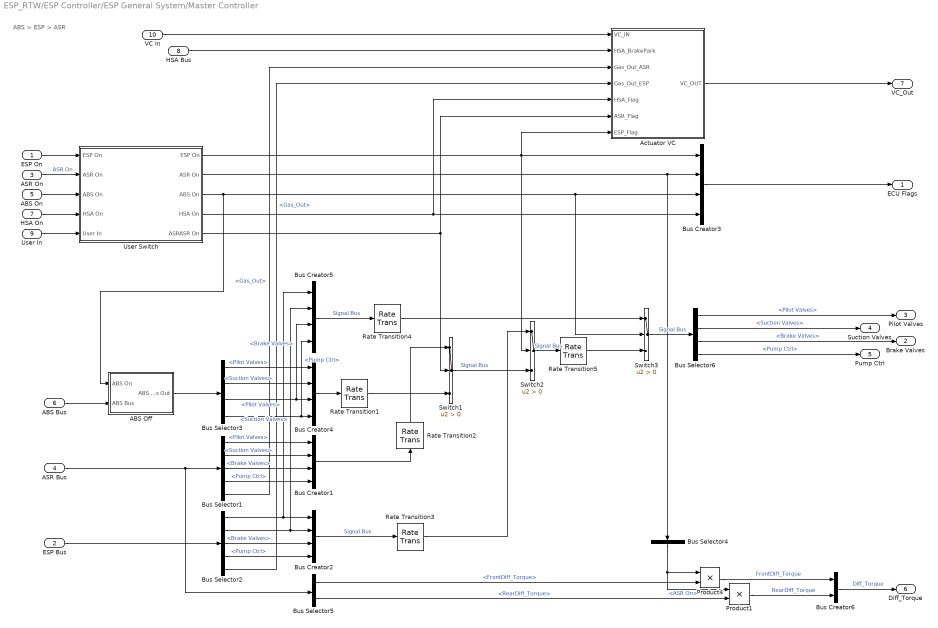
== system ESP_RTW/ESP Controller/ESP General System/Master Controller ==
  note: ABS > ESP > ASR
  ESP On : Inport
  ESP Bus : Inport  Port=2
  ASR On : Inport  Port=3
  ASR Bus : Inport  Port=4
  ABS On : Inport  Port=5
  ABS Bus : Inport  Port=6
  HSA On : Inport  Port=7
  HSA Bus : Inport  Port=8
  User In : Inport  Port=9
  VC In : Inport  Port=10
  ABS Off : Subsystem
  Actuator VC : Subsystem
  Bus Creator{1..5} (5 alike) : BusCreator  Inputs=4
  Bus Creator6 : BusCreator  Inputs=2
  Bus Selector1 : BusSelector  OutputSignals=Pilot Valves,Suction Valves,Brake Valves,Pump Ctrl,Gas_Out
  Bus Selector2 : BusSelector  OutputSignals=Pilot Valves,Suction Valves,Brake Valves,Pump Ctrl,Gas_Out
  Bus Selector3 : BusSelector  OutputSignals=Pilot Valves,Suction Valves,Brake Valves,Pump Ctrl
  Bus Selector4 : BusSelector  OutputSignals=ASR On
  Bus Selector5 : BusSelector  OutputSignals=Diff_Torque.FrontDiff_Torque,Diff_Torque.RearDiff_Torque
  Bus Selector6 : BusSelector  OutputSignals=Pilot Valves,Suction Valves,Brake Valves,Pump Ctrl
  Product1 : Product  RndMeth=Zero
  Product4 : Product  RndMeth=Zero
  Rate Transition{1..5} (5 alike) : RateTransition
  Switch1 : Switch  Criteria=u2 > Threshold
  Switch2 : Switch  Criteria=u2 > Threshold
  Switch3 : Switch  Criteria=u2 > Threshold
  User Switch : Subsystem
  ECU Flags : Outport
  Brake Valves : Outport  Port=2
  Pilot Valves : Outport  Port=3
  Suction Valves : Outport  Port=4
  Pump Ctrl : Outport  Port=5
  Diff_Torque : Outport  Port=6
  VC_Out : Outport  Port=7
  wires:
  Rate Transition5/1 -> Switch3/3
  Rate Transition4/1 -> Switch3/1
  Rate Transition3/1 -> Switch2/1
  ABS Off/1(ABS Bus Out) -> Bus Selector3/1
  Bus Selector4/1 -> Product4/1, Product1/1  "<ASR On>"
  Bus Creator6/1 -> Diff_Torque/1  "Diff_Torque"
  Product1/1 -> Bus Creator6/2  "RearDiff_Torque"
  Product4/1 -> Bus Creator6/1  "FrontDiff_Torque"
  Bus Selector5/2 -> Product1/2  "<RearDiff_Torque>"
  Bus Selector5/1 -> Product4/2  "<FrontDiff_Torque>"
  User Switch/4("HSA On ") -> Actuator VC/5(HSA_Flag), Bus Creator3/4
  HSA On/1 -> User Switch/4(HSA On)
  HSA Bus/1 -> Actuator VC/2(HSA_BrakePark)
  User Switch/2("ASR On ") -> Bus Selector4/1, Bus Creator3/2
  User In/1 -> User Switch/5(User In)
  ABS On/1 -> User Switch/3(ABS On)
  ASR On/1 -> User Switch/2(ASR On)  "ASR On"
  ESP On/1 -> User Switch/1(ESP On)
  User Switch/1("ESP On ") -> Switch2/2, Bus Creator3/1, Actuator VC/7(ESP_Flag)
  User Switch/5(ASRASR On) -> Switch1/2, Actuator VC/6(ASR_Flag)
  User Switch/3("ABS On ") -> Switch3/2, Bus Creator3/3, ABS Off/1(ABS On)
  Bus Selector2/5 -> Actuator VC/4(Gas_Out_ESP)  "<Gas_Out>"
  Bus Selector1/5 -> Actuator VC/3(Gas_Out_ASR)  "<Gas_Out>"
  Switch3/1 -> Bus Selector6/1  "Signal Bus"
  Rate Transition1/1 -> Switch1/3
  Rate Transition2/1 -> Switch1/1
  Bus Creator4/1 -> Rate Transition1/1
  Bus Creator1/1 -> Rate Transition2/1
  Bus Creator5/1 -> Rate Transition4/1  "Signal Bus"
  Switch2/1 -> Rate Transition5/1  "Signal Bus"
  Bus Selector1/4 -> Bus Creator1/4  "<Pump Ctrl>"
  Bus Selector1/3 -> Bus Creator1/3  "<Brake Valves>"
  Bus Selector1/2 -> Bus Creator1/2  "<Suction Valves>"
  Bus Selector1/1 -> Bus Creator1/1  "<Pilot Valves>"
  ASR Bus/1 -> Bus Selector1/1, Bus Selector5/1
  Bus Creator2/1 -> Rate Transition3/1  "Signal Bus"
  Switch1/1 -> Switch2/3  "Signal Bus"
  Bus Selector3/2 -> Bus Creator4/2  "<Suction Valves>"
  Bus Selector3/1 -> Bus Creator4/1  "<Pilot Valves>"
  ABS Bus/1 -> ABS Off/2(ABS Bus)
  Bus Selector3/4 -> Bus Creator4/4, Bus Creator5/4  "<Pump Ctrl>"
  Bus Selector3/3 -> Bus Creator4/3, Bus Creator5/3  "<Brake Valves>"
  Bus Selector6/4 -> Pump Ctrl/1  "<Pump Ctrl>"
  Bus Selector6/3 -> Brake Valves/1  "<Brake Valves>"
  Bus Selector6/2 -> Suction Valves/1  "<Suction Valves>"
  Bus Selector6/1 -> Pilot Valves/1  "<Pilot Valves>"
  Bus Selector2/4 -> Bus Creator2/4  "<Pump Ctrl>"
  Bus Selector2/3 -> Bus Creator2/3  "<Brake Valves>"
  Bus Selector2/2 -> Bus Creator2/2, Bus Creator5/2  "<Suction Valves>"
  Bus Selector2/1 -> Bus Creator2/1, Bus Creator5/1  "<Pilot Valves>"
  ESP Bus/1 -> Bus Selector2/1
  VC In/1 -> Actuator VC/1(VC_IN)
  Actuator VC/1(VC_OUT) -> VC_Out/1
  Bus Creator3/1 -> ECU Flags/1

== system ESP_RTW/ESP Controller/ESP General System/Signal Handling ==
  ESP In : Inport
  Vehicle Params : Inport  Port=2
  " " : simulink_extras/Transformations/Degrees to Radians
  "  " : simulink_extras/Transformations/Degrees to Radians
  "   " : Gain  Gain=RpM2RADpS
  "     " : Gain  Gain=RpM2RADpS
  "      " : Gain  Gain=RpM2RADpS
  Bus Creator : BusCreator  Inputs=4
  Bus Creator1 : BusCreator  Inputs=4
  Bus Creator2 : BusCreator  Inputs=6
  Bus Creator3 : BusCreator  Inputs=2
  Bus Creator4 : BusCreator  Inputs=2
  Bus Creator5 : BusCreator  Inputs=1
  Bus Selector1 : BusSelector  OutputSignals=WheelSpd FL [rpm],WheelSpd FR [rpm],WheelSpd RL [rpm],WheelSpd RR [rpm],Master Cylinder Pressure [bar],Throttle Valve Position [%],Sensor Longitudinal acceleration [g],Engine Speed [rpm],GearState [-],Torque Converter Speed [rpm],Sensor YawRate [degs],Steering Wheel Angle [deg],Sensor Lateral acceleration [g],Cylinder Pressure FL [bar],Cylinder Pressure FR [bar],Cylinder Pressure RL [bar],Cylinder Pressure RR [bar],Engine crankshaft output torque [Nm]
  Bus Selector2 : BusSelector  OutputSignals=SteeringGeometry
  Bus Selector3 : BusSelector  OutputSignals=SteerWheelAng_In,SteerAng_Out
  Gain2 : Gain  Gain=g  SaturateOnIntegerOverflow=on  OutDataTypeStr=Inherit: Same as input  ParamDataTypeStr=Inherit: Same as input
  Gain7 : Gain  Gain=g  SaturateOnIntegerOverflow=on  OutDataTypeStr=Inherit: Same as input  ParamDataTypeStr=Inherit: Same as input
  Lookup Table Dynamic : simulink/Lookup Tables/Lookup Table Dynamic  LookUpMeth=Interpolation-Use End Values  OutDataTypeStr=fixdt('double')  OutputDataTypeScalingMode=Specify via dialog  OutDataType=fixdt('double')  OutScaling=2^-10  DoSatur=off
  Termiator : Terminator
  Terminator1 : Terminator
  Terminator2 : Terminator
  Terminator4 : Terminator
  rpmin2rad/s : Gain  Gain=RpM2RADpS
  vquer_VA3 : Gain  Gain=0.01
  Signal Bus ESP : Outport
  Signal Bus ASR : Outport  Port=2
  Signal Bus ABS : Outport  Port=3
  Signal Bus HSA : Outport  Port=4
  wires:
  Bus Selector3/1 -> Lookup Table Dynamic/2  "<SteerWheelAng_In>"
  Bus Selector3/2 -> Lookup Table Dynamic/3  "<SteerAng_Out>"
  Bus Selector2/1 -> Bus Selector3/1  "<SteeringGeometry>"
  Vehicle Params/1 -> Bus Selector2/1
  Bus Creator5/1 -> Signal Bus HSA/1
  Bus Creator4/1 -> Signal Bus ABS/1
  Bus Selector1/18 -> Bus Creator5/1  "<Engine crankshaft output torque [Nm]>"
  Bus Creator3/1 -> Signal Bus ASR/1
  Bus Creator/1 -> Bus Creator3/1, Bus Creator4/1  "WheelSpeeds"
  Bus Creator2/1 -> Signal Bus ESP/1
  Bus Creator1/1 -> Bus Creator2/6  "Wheel Cylinder Pressure"
  Bus Selector1/14 -> Bus Creator1/1  "<Cylinder Pressure FL [bar]>"
  Bus Selector1/16 -> Bus Creator1/3  "<Cylinder Pressure RL [bar]>"
  Bus Selector1/17 -> Bus Creator1/4  "<Cylinder Pressure RR [bar]>"
  Bus Selector1/15 -> Bus Creator1/2  "<Cylinder Pressure FR [bar]>"
  vquer_VA3/1 -> Bus Creator3/2, Bus Creator2/1  "Throttle Position"
  Gain2/1 -> Bus Creator2/4  "ay [m/s^2]"
  " "/1 -> Bus Creator2/2  "Yaw Rate"
  Lookup Table Dynamic/1 -> Bus Creator2/3  "Steer Angle"
  ESP In/1 -> Bus Selector1/1
  Bus Selector1/6 -> vquer_VA3/1  "<Throttle Valve Position [%]>"
  Gain7/1 -> Bus Creator2/5, Bus Creator4/2  "ax [m/s^2]"
  "      "/1 -> Bus Creator/4  "WheelSpd_RR"
  "     "/1 -> Bus Creator/3  "WheelSpd_RL"
  "   "/1 -> Bus Creator/2  "WheelSpd_FR"
  Bus Selector1/13 -> Gain2/1  "<Sensor Lateral acceleration [g]>"
  Bus Selector1/12 -> "  "/1  "<Steering Wheel Angle [deg]>"
  Bus Selector1/11 -> " "/1  "<Sensor YawRate [degs]>"
  Bus Selector1/10 -> Termiator/1  "<Torque Converter Speed [rpm]>"
  Bus Selector1/9 -> Terminator1/1  "<GearState [-]>"
  Bus Selector1/8 -> Terminator2/1  "<Engine Speed [rpm]>"
  Bus Selector1/5 -> Terminator4/1  "<Master Cylinder Pressure [bar]>"
  Bus Selector1/7 -> Gain7/1  "<Sensor Longitudinal acceleration [g]>"
  Bus Selector1/4 -> "      "/1  "<WheelSpd RR [rpm]>"
  Bus Selector1/3 -> "     "/1  "<WheelSpd RL [rpm]>"
  Bus Selector1/2 -> "   "/1  "<WheelSpd FR [rpm]>"
  Bus Selector1/1 -> rpmin2rad/s/1  "<WheelSpd FL [rpm]>"
  rpmin2rad/s/1 -> Bus Creator/1  "WheelSpd_FL"
  "  "/1 -> Lookup Table Dynamic/1
